simulink model "trng_controller_circuit_level"  (R2024a)
settings: Solver=VariableStepAuto  StartTime=0.0  StopTime=50  RelTol=1e-3
undefined symbols (not defined in the file or in its folder): band_width, C1, R, tpulse
libraries: simulink x5, slpidlib x2
settings Model: Creator=manik  LastModifiedBy=manik

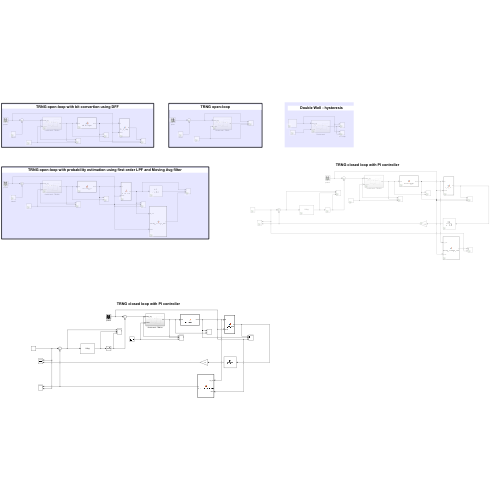
[thumbnail: Simulink's stored preview of the top-level diagram]
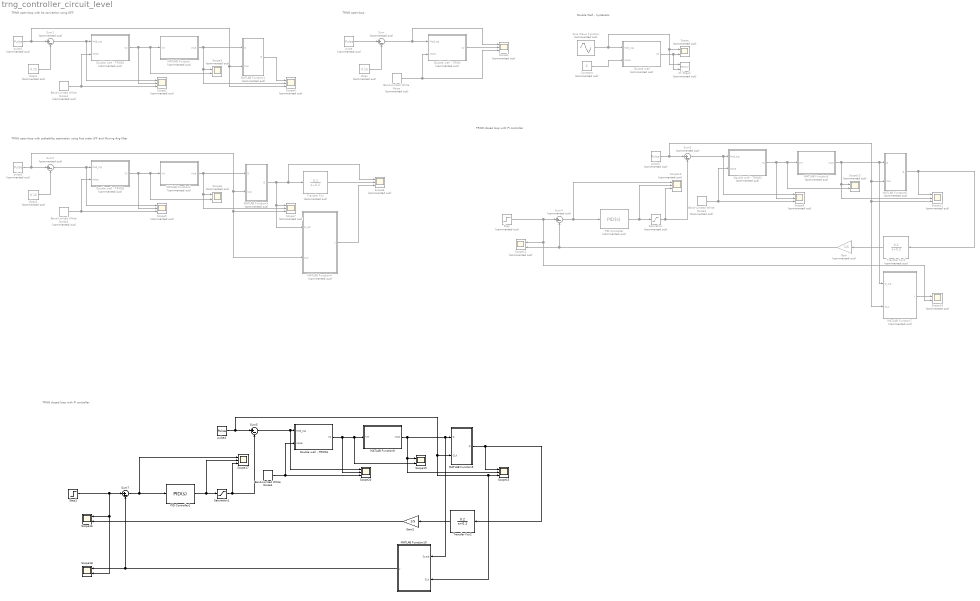
== system trng_controller_circuit_level ==
  note: TRNG open-loop
  note: Double Well - hysteresis
  note: TRNG open-loop with bit convertion using DFF
  note: TRNG open-loop with probability estimation using first order LPF and Moving Avg filter
  note: TRNG closed loop with PI controller
  note: TRNG closed loop with PI controller
  Band-Limited White Noise : simulink/Sources/Band-Limited White Noise  Commented=on  Cov=[0.000005]  Ts=1/band_width  seed=[23341]
  Band-Limited White Noise1 : simulink/Sources/Band-Limited White Noise  Commented=on  Cov=[0.000005]  Ts=1/band_width  seed=[23341]
  Band-Limited White Noise2 : simulink/Sources/Band-Limited White Noise  Commented=on  Cov=[0.000005]  Ts=1/band_width  seed=[23341]
  Band-Limited White Noise3 : simulink/Sources/Band-Limited White Noise  Commented=on  Cov=[0.000005]  Ts=1/80e3  seed=[23341]
  Band-Limited White Noise4 : simulink/Sources/Band-Limited White Noise  Cov=[0.00001]  Ts=1/80e3  seed=[23341]
  Constant : Constant  Commented=on  Value=0
  Double well : Subsystem  Commented=on
  Double well - TRNG : Subsystem  Commented=on
  Double well - TRNG1 : Subsystem  Commented=on
  Double well - TRNG2 : Subsystem  Commented=on
  Double well - TRNG3 : Subsystem  Commented=on
  Double well - TRNG4 : Subsystem
  Gain : Gain  Commented=on  Gain=1/5
  Gain2 : Gain  Gain=1/5
  MATLAB Function : MATLAB Function  Commented=on  TreatAsAtomicUnit=on
  MATLAB Function1 : MATLAB Function  Commented=on  TreatAsAtomicUnit=on
  MATLAB Function10 : MATLAB Function  TreatAsAtomicUnit=on
  MATLAB Function2 : MATLAB Function  Commented=on  TreatAsAtomicUnit=on
  MATLAB Function3 : MATLAB Function  Commented=on  TreatAsAtomicUnit=on
  MATLAB Function4 : MATLAB Function  Commented=on  TreatAsAtomicUnit=on
  MATLAB Function5 : MATLAB Function  Commented=on  TreatAsAtomicUnit=on
  MATLAB Function6 : MATLAB Function  Commented=on  TreatAsAtomicUnit=on
  MATLAB Function7 : MATLAB Function  Commented=on  TreatAsAtomicUnit=on
  MATLAB Function8 : MATLAB Function  TreatAsAtomicUnit=on
  MATLAB Function9 : MATLAB Function  TreatAsAtomicUnit=on
  PID Controller : slpidlib/PID Controller  Commented=on  Controller=PID  Form=Parallel  TimeDomain=Continuous-time  UseExternalTs=off  SampleTime=-1  IntegratorMethod=Forward Euler  FilterMethod=Forward Euler  ControllerParametersSource=internal  P=1  I=0.5  UseKiTs=off  D=0.1  UseExternalDerivativeSource=off  N=100  UseFilter=on  TunerSelectOption=Transfer Function Based (PID Tuner App)  InitialConditionSource=internal  InitialConditionForIntegrator=0  InitialConditionForFilter=0  DifferentiatorICPrevScaledInput=0  ExternalReset=none  TrackingMode=off  Kt=1  LimitOutput=off  SatLimitsSource=internal  UpperSaturationLimit=inf  LowerSaturationLimit=-inf  LinearizeAsGain=on  AntiWindupMode=none  Kb=1  LimitIntegrator=off  UpperIntegratorSaturationLimit=inf  LowerIntegratorSaturationLimit=-inf  POutMin=[]  POutMax=[]  IOutMin=[]  IOutMax=[]  DOutMin=[]  DOutMax=[]  NOutMin=[]  NOutMax=[]  SumOutMin=[]  SumOutMax=[]  SaturationOutMin=[]  SaturationOutMax=[]  PParamMin=[]  PParamMax=[]  IParamMin=[]  IParamMax=[]  DParamMin=[]  DParamMax=[]  NParamMin=[]  NParamMax=[]  KbParamMin=[]  KbParamMax=[]  KtParamMin=[]  KtParamMax=[]  KbOutMin=[]  KbOutMax=[]  KtOutMin=[]  KtOutMax=[]  IntegratorOutMin=[]  IntegratorOutMax=[]  FilterOutMin=[]  FilterOutMax=[]  SumI1OutMin=[]  SumI1OutMax=[]  SumI2OutMin=[]  SumI2OutMax=[]  SumI3OutMin=[]  SumI3OutMax=[]  SumI4OutMin=[]  SumI4OutMax=[]  SumDOutMin=[]  SumDOutMax=[]  DifferentiatorOutMin=[]  DifferentiatorOutMax=[]  FilterDiffOutCoefMin=[]  FilterDiffOutCoefMax=[]  ReciprocalOutMin=[]  ReciprocalOutMax=[]  SumDenOutMin=[]  SumDenOutMax=[]  SumNumOutMin=[]  SumNumOutMax=[]  DivideOutMin=[]  DivideOutMax=[]  UdiffTsProdOutMin=[]  UdiffTsProdOutMax=[]  NTsProdOutMin=[]  NTsProdOutMax=[]  UintegralTsProdOutMin=[]  UintegralTsProdOutMax=[]  UngainTsProdOutMin=[]  UngainTsProdOutMax=[]  ClampingZeroOutDataTypeStr=Inherit: Inherit via back propagation  ClampingZeroOutMin=[]  ClampingZeroOutMax=[]  FilterDenConstantOutDataTypeStr=Inherit: Inherit via back propagation  FilterDenConstantOutMin=[]  FilterDenConstantOutMax=[]  PCopyOutDataTypeStr=Inherit: Inherit via back propagation  PCopyOutMin=[]  PCopyOutMax=[]  NCopyOutDataTypeStr=Inherit: Inherit via back propagation  NCopyOutMin=[]  NCopyOutMax=[]  IntegratorContinuousStateAttributes=''  IntegratorStateMustResolveToSignalObject=off  IntegratorRTWStateStorageClass=Auto  FilterContinuousStateAttributes=''  FilterStateMustResolveToSignalObject=off  FilterRTWStateStorageClass=Auto  ParallelPVariant=InternalParameters  IdealPVariant=Disabled  IVariant=InternalParameters  DVariant=InternalParameters  IntegratorVariant=Continuous  SatVariant=Disabled  AWVariant=Passthrough  PCopyVariant=Disabled  TRVariant=Disabled  FdbkBlocksVariant=Forward  IdealPFdbkVariant=Disabled  SatFdbkVariant=Disabled  DerivativeFilterVariant=ContFilter  NVariant=InternalParameters  NCopyVariant=Disabled  FilterICVariant=InternalICsFilter  IntegratorICVariant=InternalICs  ExternalResetVariant=Disabled  TRSumVariant=Passthrough  SumFdbkVariant=Disabled  SumVariant=Sum_PID  TsampFilterVariant=InternalTs  TsampNgainVariant=Passthrough  TsampIntegralVariant=Disabled_SignalSpec  ExternalSaturationOutDataTypeStr=Inherit: Same as second input  DerivativeSourceVariant=ErrorSignal
  PID Controller1 : slpidlib/PID Controller  Controller=PID  Form=Parallel  TimeDomain=Continuous-time  UseExternalTs=off  SampleTime=-1  IntegratorMethod=Forward Euler  FilterMethod=Forward Euler  ControllerParametersSource=internal  P=1  I=0.5  UseKiTs=off  D=0.1  UseExternalDerivativeSource=off  N=100  UseFilter=on  TunerSelectOption=Transfer Function Based (PID Tuner App)  InitialConditionSource=internal  InitialConditionForIntegrator=0  InitialConditionForFilter=0  DifferentiatorICPrevScaledInput=0  ExternalReset=none  TrackingMode=off  Kt=1  LimitOutput=off  SatLimitsSource=internal  UpperSaturationLimit=inf  LowerSaturationLimit=-inf  LinearizeAsGain=on  AntiWindupMode=none  Kb=1  LimitIntegrator=off  UpperIntegratorSaturationLimit=inf  LowerIntegratorSaturationLimit=-inf  POutMin=[]  POutMax=[]  IOutMin=[]  IOutMax=[]  DOutMin=[]  DOutMax=[]  NOutMin=[]  NOutMax=[]  SumOutMin=[]  SumOutMax=[]  SaturationOutMin=[]  SaturationOutMax=[]  PParamMin=[]  PParamMax=[]  IParamMin=[]  IParamMax=[]  DParamMin=[]  DParamMax=[]  NParamMin=[]  NParamMax=[]  KbParamMin=[]  KbParamMax=[]  KtParamMin=[]  KtParamMax=[]  KbOutMin=[]  KbOutMax=[]  KtOutMin=[]  KtOutMax=[]  IntegratorOutMin=[]  IntegratorOutMax=[]  FilterOutMin=[]  FilterOutMax=[]  SumI1OutMin=[]  SumI1OutMax=[]  SumI2OutMin=[]  SumI2OutMax=[]  SumI3OutMin=[]  SumI3OutMax=[]  SumI4OutMin=[]  SumI4OutMax=[]  SumDOutMin=[]  SumDOutMax=[]  DifferentiatorOutMin=[]  DifferentiatorOutMax=[]  FilterDiffOutCoefMin=[]  FilterDiffOutCoefMax=[]  ReciprocalOutMin=[]  ReciprocalOutMax=[]  SumDenOutMin=[]  SumDenOutMax=[]  SumNumOutMin=[]  SumNumOutMax=[]  DivideOutMin=[]  DivideOutMax=[]  UdiffTsProdOutMin=[]  UdiffTsProdOutMax=[]  NTsProdOutMin=[]  NTsProdOutMax=[]  UintegralTsProdOutMin=[]  UintegralTsProdOutMax=[]  UngainTsProdOutMin=[]  UngainTsProdOutMax=[]  ClampingZeroOutDataTypeStr=Inherit: Inherit via back propagation  ClampingZeroOutMin=[]  ClampingZeroOutMax=[]  FilterDenConstantOutDataTypeStr=Inherit: Inherit via back propagation  FilterDenConstantOutMin=[]  FilterDenConstantOutMax=[]  PCopyOutDataTypeStr=Inherit: Inherit via back propagation  PCopyOutMin=[]  PCopyOutMax=[]  NCopyOutDataTypeStr=Inherit: Inherit via back propagation  NCopyOutMin=[]  NCopyOutMax=[]  IntegratorContinuousStateAttributes=''  IntegratorStateMustResolveToSignalObject=off  IntegratorRTWStateStorageClass=Auto  FilterContinuousStateAttributes=''  FilterStateMustResolveToSignalObject=off  FilterRTWStateStorageClass=Auto  ParallelPVariant=InternalParameters  IdealPVariant=Disabled  IVariant=InternalParameters  DVariant=InternalParameters  IntegratorVariant=Continuous  SatVariant=Disabled  AWVariant=Passthrough  PCopyVariant=Disabled  TRVariant=Disabled  FdbkBlocksVariant=Forward  IdealPFdbkVariant=Disabled  SatFdbkVariant=Disabled  DerivativeFilterVariant=ContFilter  NVariant=InternalParameters  NCopyVariant=Disabled  FilterICVariant=InternalICsFilter  IntegratorICVariant=InternalICs  ExternalResetVariant=Disabled  TRSumVariant=Passthrough  SumFdbkVariant=Disabled  SumVariant=Sum_PID  TsampFilterVariant=InternalTs  TsampNgainVariant=Passthrough  TsampIntegralVariant=Disabled_SignalSpec  ExternalSaturationOutDataTypeStr=Inherit: Same as second input  DerivativeSourceVariant=ErrorSignal
  Saturation : Saturate  Commented=on  UpperLimit=0.25  LowerLimit=0
  Saturation1 : Saturate  UpperLimit=0.25  LowerLimit=0
  Scope{,3,6,10,12,14} (6 alike) : Scope  Commented=on  NumInputPorts=2
  Scope{1..2,4..5,7..9,11,13} (9 alike) : Scope  Commented=on  NumInputPorts=3
  Scope15 : Scope  NumInputPorts=3
  Scope16 : Scope  NumInputPorts=2
  Scope17 : Scope  NumInputPorts=3
  Scope18 : Scope  NumInputPorts=2
  Scope19 : Scope  NumInputPorts=2
  Scope20 : Scope  NumInputPorts=3
  Sine Wave Function : Sin  Commented=on  Amplitude=5  SampleTime=0
  Step : Step  Commented=on  Time=20  Before=0.4  After=0.6  SampleTime=0
  Step1 : Step  Time=20  Before=0.4  After=0.6  SampleTime=0
  Sum{,1..4} (5 alike) : Sum  Commented=on  Inputs=|+-
  Sum5 : Sum  Inputs=|+-
  Sum7 : Sum  Inputs=|+-
  Transfer Fcn : TransferFcn  Commented=on  Numerator=[0.2]  Denominator=[1 0.2]
  Transfer Fcn1 : TransferFcn  Commented=on  Numerator=[0.2]  Denominator=[1 0.2]
  Transfer Fcn2 : TransferFcn  Numerator=[0.2]  Denominator=[1 0.2]
  Vbias : Constant  Commented=on  Value=0.15
  Vbias1 : Constant  Commented=on  Value=0.15
  Vbias2 : Constant  Commented=on  Value=0.15
  XY Graph : Record  Commented=on  FileSettingsInternal="{\"entries\":[{\"content\":{\"excelSettings\":{\"content\":{},\"type\":\"Streamout.ExcelSettings\"}},\"type\":\"Streamout.FileSettingStorage\",\"uuid\":\"\"}],\"packageUris\":[\"http:\\/\\/schema.mathworks.com\\/mf0\\/streamout_blocks\\/R2020a\"],\"version\":\"1.0\"}"  Layout=[1 1]  SignalsInternal="{\"entries\":[{\"content\":{},\"type\":\"RecordBlkView.InputSignals\",\"uuid\":\"\"}],\"packageUris\":[\"http:\\/\\/schema.mathworks.com\\/mf0\\/streamout_blocks\\/R2020a\"],\"version\":\"1.0\"}"  VisualizationBindings="{\"xyplotplugin\":{\"info\":[{\"series\":[],\"subplotID\":1}]}}"  CompatibilityTag=XY
  pulse : DiscretePulseGenerator  Commented=on  PulseType=Time based  Amplitude=5  Period=tpulse  PulseWidth=50
  pulse1 : DiscretePulseGenerator  Commented=on  PulseType=Time based  Amplitude=5  Period=tpulse  PulseWidth=50
  pulse2 : DiscretePulseGenerator  Commented=on  PulseType=Time based  Amplitude=5  Period=tpulse  PulseWidth=50
  pulse3 : DiscretePulseGenerator  Commented=on  PulseType=Time based  Amplitude=5  Period=20e-3  PulseWidth=50
  pulse4 : DiscretePulseGenerator  PulseType=Time based  Amplitude=5  Period=20e-3  PulseWidth=50
  wires:
  Sine Wave Function/1 -> XY Graph/1, Scope/1, Double well/1(Mod_sig)
  Constant/1 -> Double well/2(noise)
  Double well/1(V2) -> XY Graph/2, Scope/2
  pulse/1 -> Sum/1
  Vbias/1 -> Sum/2
  Sum/1 -> Scope1/1, Double well - TRNG/1(Mod_sig)
  Double well - TRNG/1(V2) -> Scope1/2
  Band-Limited White Noise/1 -> Scope1/3, Double well - TRNG/2(noise)
  Double well - TRNG1/1(V2) -> Scope2/2, Scope3/2, MATLAB Function/1(Vin)
  Vbias1/1 -> Sum1/2
  Band-Limited White Noise1/1 -> Double well - TRNG1/2(noise), Scope2/3
  Sum1/1 -> Double well - TRNG1/1(Mod_sig), Scope2/1
  pulse1/1 -> Scope4/3, MATLAB Function1/2(CLK), Sum1/1
  MATLAB Function/1(Vout) -> MATLAB Function1/1(D), Scope3/1, Scope4/2
  MATLAB Function1/1(Q) -> Scope4/1
  pulse2/1 -> MATLAB Function4/2(CLK), Scope7/3, MATLAB Function3/2(CLK), Sum2/1
  Sum2/1 -> Double well - TRNG2/1(Mod_sig), Scope5/1
  Band-Limited White Noise2/1 -> Double well - TRNG2/2(noise), Scope5/3
  Vbias2/1 -> Sum2/2
  Double well - TRNG2/1(V2) -> Scope5/2, Scope6/2, MATLAB Function2/1(Vin)
  MATLAB Function3/1(Q) -> Scope8/1, Transfer Fcn/1, MATLAB Function4/1(D_out), Scope7/1
  MATLAB Function2/1(Vout) -> MATLAB Function3/1(D), Scope6/1, Scope7/2
  Transfer Fcn/1 -> Scope8/2
  MATLAB Function4/1(y) -> Scope8/3
  MATLAB Function6/1(Q) -> Scope11/1, Transfer Fcn1/1
  MATLAB Function5/1(Vout) -> MATLAB Function7/1(D_out), MATLAB Function6/1(D), Scope10/1, Scope11/2
  Band-Limited White Noise3/1 -> Double well - TRNG3/2(noise), Scope9/3
  Sum3/1 -> Double well - TRNG3/1(Mod_sig), Scope9/1
  pulse3/1 -> MATLAB Function7/2(CLK), Scope11/3, MATLAB Function6/2(CLK), Sum3/1
  Double well - TRNG3/1(V2) -> Scope9/2, Scope10/2, MATLAB Function5/1(Vin)
  Transfer Fcn1/1 -> Gain/1
  Gain/1 -> Scope12/2, Sum4/2
  Step/1 -> Scope14/2, Scope12/1, Sum4/1
  Sum4/1 -> PID Controller/1, Scope13/1
  PID Controller/1 -> Scope13/2, Saturation/1
  Saturation/1 -> Sum3/2, Scope13/3
  MATLAB Function7/1(y) -> Scope14/1
  MATLAB Function9/1(Q) -> Scope15/1, Transfer Fcn2/1
  pulse4/1 -> MATLAB Function10/2(CLK), Scope15/3, MATLAB Function9/2(CLK), Sum5/1
  MATLAB Function8/1(Vout) -> MATLAB Function10/1(D_out), MATLAB Function9/1(D), Scope19/1, Scope15/2
  Sum5/1 -> Double well - TRNG4/1(Mod_sig), Scope20/1
  Transfer Fcn2/1 -> Gain2/1
  Double well - TRNG4/1(V2) -> Scope20/2, Scope19/2, MATLAB Function8/1(Vin)
  Step1/1 -> Scope18/2, Scope16/1, Sum7/1
  Saturation1/1 -> Sum5/2, Scope17/3
  PID Controller1/1 -> Scope17/2, Saturation1/1
  MATLAB Function10/1(y) -> Sum7/2, Scope18/1
  Band-Limited White Noise4/1 -> Double well - TRNG4/2(noise), Scope20/3
  Sum7/1 -> PID Controller1/1, Scope17/1
  Gain2/1 -> Scope16/2

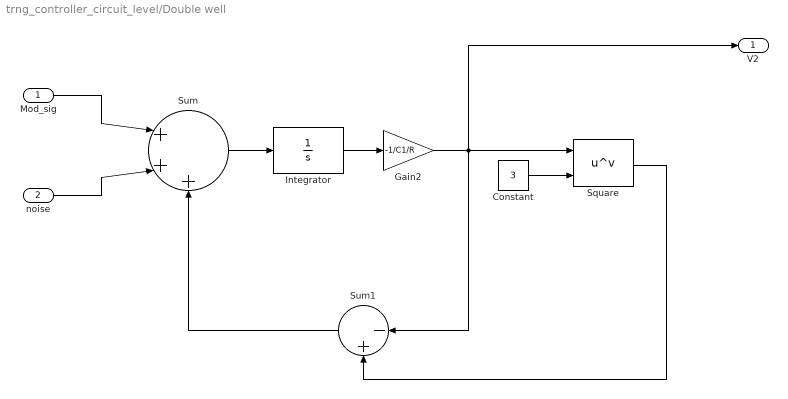
== system trng_controller_circuit_level/Double well ==
  Mod_sig : Inport
  noise : Inport  Port=2
  Constant : Constant  Value=3
  Gain2 : Gain  Gain=-1/C1/R
  Integrator : Integrator
  Square : Math  Operator=pow
  Sum : Sum  Inputs=|+++
  Sum1 : Sum  Inputs=|-+
  V2 : Outport
  wires:
  Sum/1 -> Integrator/1
  Integrator/1 -> Gain2/1
  Gain2/1 -> V2/1, Square/1, Sum1/1
  Constant/1 -> Square/2
  Square/1 -> Sum1/2
  noise/1 -> Sum/2
  Mod_sig/1 -> Sum/1
  Sum1/1 -> Sum/3

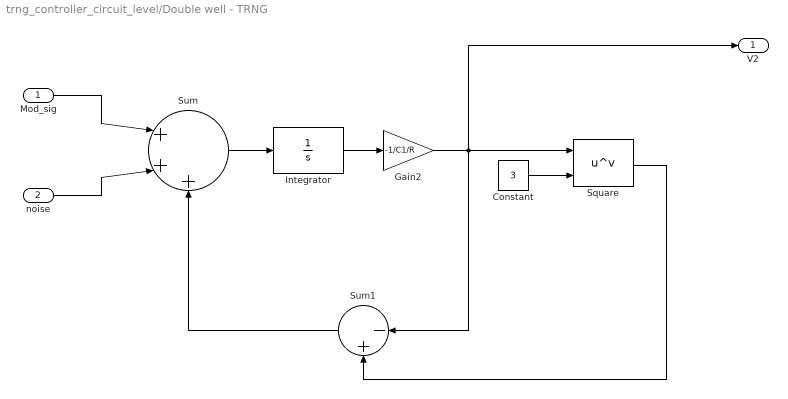
== system trng_controller_circuit_level/Double well - TRNG ==
  Mod_sig : Inport
  noise : Inport  Port=2
  Constant : Constant  Value=3
  Gain2 : Gain  Gain=-1/C1/R
  Integrator : Integrator
  Square : Math  Operator=pow
  Sum : Sum  Inputs=|+++
  Sum1 : Sum  Inputs=|-+
  V2 : Outport
  wires:
  Sum/1 -> Integrator/1
  Integrator/1 -> Gain2/1
  Gain2/1 -> V2/1, Square/1, Sum1/1
  Constant/1 -> Square/2
  Square/1 -> Sum1/2
  noise/1 -> Sum/2
  Mod_sig/1 -> Sum/1
  Sum1/1 -> Sum/3

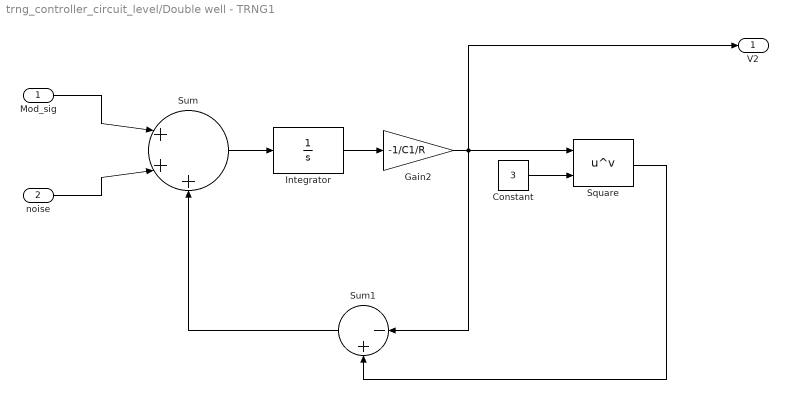
== system trng_controller_circuit_level/Double well - TRNG1 ==
  Mod_sig : Inport
  noise : Inport  Port=2
  Constant : Constant  Value=3
  Gain2 : Gain  Gain=-1/C1/R
  Integrator : Integrator
  Square : Math  Operator=pow
  Sum : Sum  Inputs=|+++
  Sum1 : Sum  Inputs=|-+
  V2 : Outport
  wires:
  Sum/1 -> Integrator/1
  Integrator/1 -> Gain2/1
  Gain2/1 -> V2/1, Square/1, Sum1/1
  Constant/1 -> Square/2
  Square/1 -> Sum1/2
  noise/1 -> Sum/2
  Mod_sig/1 -> Sum/1
  Sum1/1 -> Sum/3

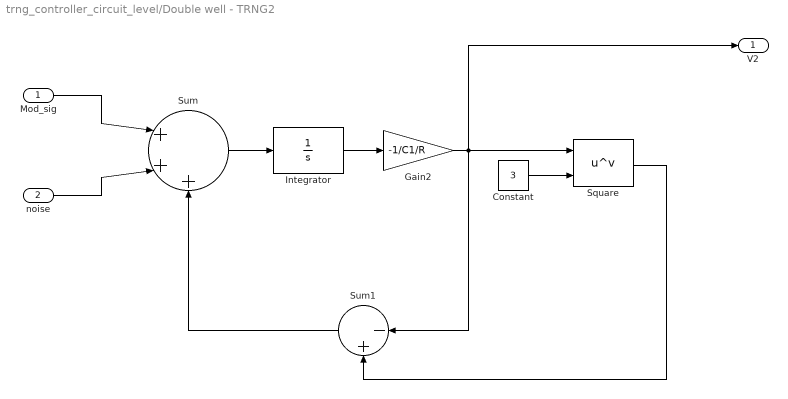
== system trng_controller_circuit_level/Double well - TRNG2 ==
  Mod_sig : Inport
  noise : Inport  Port=2
  Constant : Constant  Value=3
  Gain2 : Gain  Gain=-1/C1/R
  Integrator : Integrator
  Square : Math  Operator=pow
  Sum : Sum  Inputs=|+++
  Sum1 : Sum  Inputs=|-+
  V2 : Outport
  wires:
  Sum/1 -> Integrator/1
  Integrator/1 -> Gain2/1
  Gain2/1 -> V2/1, Square/1, Sum1/1
  Constant/1 -> Square/2
  Square/1 -> Sum1/2
  noise/1 -> Sum/2
  Mod_sig/1 -> Sum/1
  Sum1/1 -> Sum/3

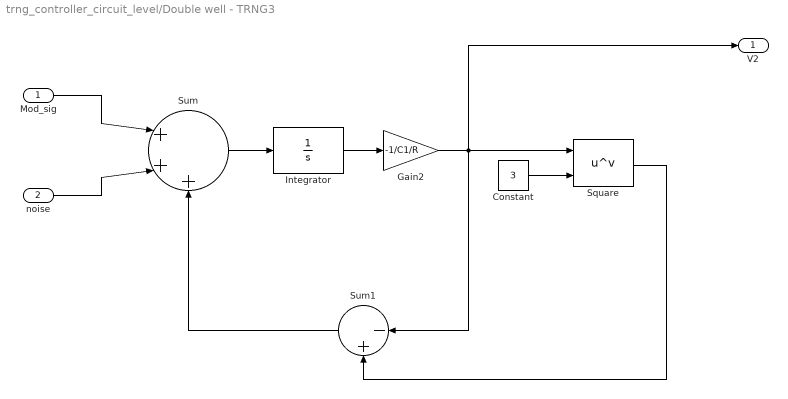
== system trng_controller_circuit_level/Double well - TRNG3 ==
  Mod_sig : Inport
  noise : Inport  Port=2
  Constant : Constant  Value=3
  Gain2 : Gain  Gain=-1/C1/R
  Integrator : Integrator
  Square : Math  Operator=pow
  Sum : Sum  Inputs=|+++
  Sum1 : Sum  Inputs=|-+
  V2 : Outport
  wires:
  Sum/1 -> Integrator/1
  Integrator/1 -> Gain2/1
  Gain2/1 -> V2/1, Square/1, Sum1/1
  Constant/1 -> Square/2
  Square/1 -> Sum1/2
  noise/1 -> Sum/2
  Mod_sig/1 -> Sum/1
  Sum1/1 -> Sum/3

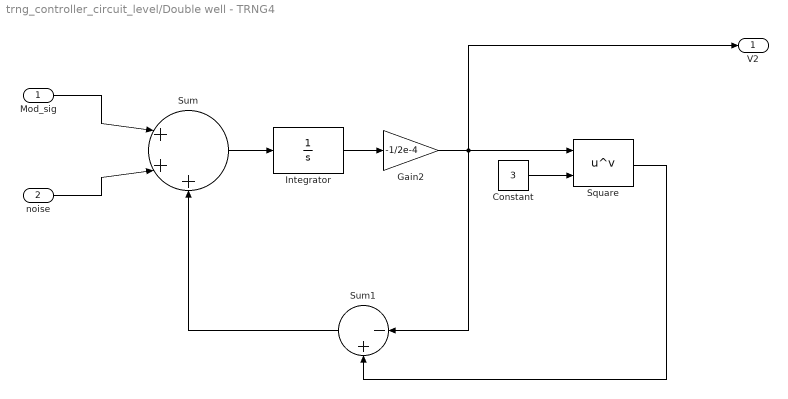
== system trng_controller_circuit_level/Double well - TRNG4 ==
  Mod_sig : Inport
  noise : Inport  Port=2
  Constant : Constant  Value=3
  Gain2 : Gain  Gain=-1/2e-4
  Integrator : Integrator
  Square : Math  Operator=pow
  Sum : Sum  Inputs=|+++
  Sum1 : Sum  Inputs=|-+
  V2 : Outport
  wires:
  Sum/1 -> Integrator/1
  Integrator/1 -> Gain2/1
  Gain2/1 -> V2/1, Square/1, Sum1/1
  Constant/1 -> Square/2
  Square/1 -> Sum1/2
  noise/1 -> Sum/2
  Mod_sig/1 -> Sum/1
  Sum1/1 -> Sum/3

== matlab function trng_controller_circuit_level/MATLAB Function ==
  settings: updateMethod=DISCRETE
  data: Vin input; Vout output
function Vout = schmittTrigger(Vin)
% u is the input signal
% y is the output signal

% Define thresholds
V_high = 0.75;
V_low = -0.75;

% Define output states
output_high = 5;
output_low = 0;

% Declare a persistent variable for the state
persistent state;
if isempty(state)
    state = output_low; % Initialize state
end

% Implement Schmitt trigger logic
if Vin > V_high
    state = output_high;
elseif Vin < V_low
    state = output_low;
end

% Output the current state
Vout = state;
end

== matlab function trng_controller_circuit_level/MATLAB Function2 ==
  settings: updateMethod=DISCRETE
  data: Vin input; Vout output
function Vout = schmittTrigger(Vin)
% u is the input signal
% y is the output signal

% Define thresholds
V_high = 0.75;
V_low = -0.75;

% Define output states
output_high = 5;
output_low = 0;

% Declare a persistent variable for the state
persistent state;
if isempty(state)
    state = output_low; % Initialize state
end

% Implement Schmitt trigger logic
if Vin > V_high
    state = output_high;
elseif Vin < V_low
    state = output_low;
end

% Output the current state
Vout = state;
end

== matlab function trng_controller_circuit_level/MATLAB Function3 ==
  data: D input; Q output; CLK input
function Q = D_flip_flop(D, CLK)
clk_high = 5;
% D - Data input (0 or 1)
% CLK - Clock signal (should toggle between 0 and 1)

% Output Q - Flip-flop output

% Persistent variable to hold the state
persistent Q_state;
if isempty(Q_state)
    Q_state = 0; % Initial state is 0
end

% Persistent variable to detect rising edge of CLK
persistent last_CLK;
if isempty(last_CLK)
    last_CLK = 0; % Initial clock state
end

% Rising edge detection and D flip-flop logic
if (last_CLK == 0) && (CLK == clk_high)
    % On rising edge of CLK, set Q to D
    Q_state = D;
end

% Update last clock state
last_CLK = CLK;

% Output the state
Q = Q_state;
end

== matlab function trng_controller_circuit_level/MATLAB Function4 ==
  data: D_out input; y output; CLK input
function y = moving_average_filter(D_out, CLK)
% D_out - Input from the D flip-flop output
% CLK - Clock signal
% y - Output after moving average filtering

% Parameters
N = 100; % Window size for moving average filter

% Persistent buffer for moving average filter and clock state
persistent buffer;
persistent last_CLK;
if isempty(buffer)
    buffer = zeros(1, N); % Initialize buffer with zeros
end
if isempty(last_CLK)
    last_CLK = 0; % Initialize last clock state
end

% Check for rising edge of the clock
if (last_CLK == 0) && (CLK == 5)
    % On rising edge of CLK, update buffer with new D_out value
    buffer = [buffer(2:end), D_out];
end

% Update last clock state
last_CLK = CLK;

% Calculate the moving average
y = mean(buffer);
end

== matlab function trng_controller_circuit_level/MATLAB Function5 ==
  settings: updateMethod=DISCRETE
  data: Vin input; Vout output
function Vout = schmittTrigger(Vin)
% u is the input signal
% y is the output signal

% Define thresholds
V_high = 0.75;
V_low = -0.75;

% Define output states
output_high = 5;
output_low = 0;

% Declare a persistent variable for the state
persistent state;
if isempty(state)
    state = output_low; % Initialize state
end

% Implement Schmitt trigger logic
if Vin > V_high
    state = output_high;
elseif Vin < V_low
    state = output_low;
end

% Output the current state
Vout = state;
end

== matlab function trng_controller_circuit_level/MATLAB Function6 ==
  data: D input; Q output; CLK input
function Q = D_flip_flop(D, CLK)
clk_high = 5;
% D - Data input (0 or 1)
% CLK - Clock signal (should toggle between 0 and 1)

% Output Q - Flip-flop output

% Persistent variable to hold the state
persistent Q_state;
if isempty(Q_state)
    Q_state = 0; % Initial state is 0
end

% Persistent variable to detect rising edge of CLK
persistent last_CLK;
if isempty(last_CLK)
    last_CLK = 0; % Initial clock state
end

% Rising edge detection and D flip-flop logic
if (last_CLK == 0) && (CLK == clk_high)
    % On rising edge of CLK, set Q to D
    Q_state = D;
end

% Update last clock state
last_CLK = CLK;

% Output the state
Q = Q_state;
end

== matlab function trng_controller_circuit_level/MATLAB Function7 ==
  data: D_out input; y output; CLK input
function y = moving_average_filter(D_out, CLK)
% D_out - Input from the D flip-flop output
% CLK - Clock signal
% y - Output after moving average filtering

% Parameters
N = 100; % Window size for moving average filter

% Persistent buffer for moving average filter and clock state
persistent buffer;
persistent last_CLK;
if isempty(buffer)
    buffer = zeros(1, N); % Initialize buffer with zeros
end
if isempty(last_CLK)
    last_CLK = 0; % Initialize last clock state
end

% Check for rising edge of the clock
if (last_CLK == 0) && (CLK == 5)
    % On rising edge of CLK, update buffer with new D_out value
    buffer = [buffer(2:end), D_out];
end

% Update last clock state
last_CLK = CLK;

% Calculate the moving average
y = mean(buffer)/5;
end

== matlab function trng_controller_circuit_level/MATLAB Function10 ==
  data: D_out input; y output; CLK input
function y = moving_average_filter(D_out, CLK)
% D_out - Input from the D flip-flop output
% CLK - Clock signal
% y - Output after moving average filtering

% Parameters
N = 100; % Window size for moving average filter

% Persistent buffer for moving average filter and clock state
persistent buffer;
persistent last_CLK;
if isempty(buffer)
    buffer = zeros(1, N); % Initialize buffer with zeros
end
if isempty(last_CLK)
    last_CLK = 0; % Initialize last clock state
end

% Check for rising edge of the clock
if (last_CLK == 0) && (CLK == 5)
    % On rising edge of CLK, update buffer with new D_out value
    buffer = [buffer(2:end), D_out];
end

% Update last clock state
last_CLK = CLK;

% Calculate the moving average
y = mean(buffer)/5;
end

== matlab function trng_controller_circuit_level/MATLAB Function8 ==
  settings: updateMethod=DISCRETE
  data: Vin input; Vout output
function Vout = schmittTrigger(Vin)
% u is the input signal
% y is the output signal

% Define thresholds
V_high = 0.75;
V_low = -0.75;

% Define output states
output_high = 5;
output_low = 0;

% Declare a persistent variable for the state
persistent state;
if isempty(state)
    state = output_low; % Initialize state
end

% Implement Schmitt trigger logic
if Vin > V_high
    state = output_high;
elseif Vin < V_low
    state = output_low;
end

% Output the current state
Vout = state;
end

== matlab function trng_controller_circuit_level/MATLAB Function1 ==
  data: D input; Q output; CLK input
function Q = D_flip_flop(D, CLK)
clk_high = 5;
% D - Data input (0 or 1)
% CLK - Clock signal (should toggle between 0 and 1)

% Output Q - Flip-flop output

% Persistent variable to hold the state
persistent Q_state;
if isempty(Q_state)
    Q_state = 0; % Initial state is 0
end

% Persistent variable to detect rising edge of CLK
persistent last_CLK;
if isempty(last_CLK)
    last_CLK = 0; % Initial clock state
end

% Rising edge detection and D flip-flop logic
if (last_CLK == 0) && (CLK == clk_high)
    % On rising edge of CLK, set Q to D
    Q_state = D;
end

% Update last clock state
last_CLK = CLK;

% Output the state
Q = Q_state;
end

== matlab function trng_controller_circuit_level/MATLAB Function9 ==
  data: D input; Q output; CLK input
function Q = D_flip_flop(D, CLK)
clk_high = 5;
% D - Data input (0 or 1)
% CLK - Clock signal (should toggle between 0 and 1)

% Output Q - Flip-flop output

% Persistent variable to hold the state
persistent Q_state;
if isempty(Q_state)
    Q_state = 0; % Initial state is 0
end

% Persistent variable to detect rising edge of CLK
persistent last_CLK;
if isempty(last_CLK)
    last_CLK = 0; % Initial clock state
end

% Rising edge detection and D flip-flop logic
if (last_CLK == 0) && (CLK == clk_high)
    % On rising edge of CLK, set Q to D
    Q_state = D;
end

% Update last clock state
last_CLK = CLK;

% Output the state
Q = Q_state;
end
